simulink model "main_table_model"  (R2013a)
settings: Solver=ode3  StartTime=0.0  StopTime=Inf  FixedStep=1/30  RelTol=1e-3
undefined symbols (not defined in the file or in its folder): gray, none, serial, strel, videoinput
libraries: simulink x5, visiontextngfix x2, visionsinks x2, instrumentlib x2, visionstatistics x1, imaqlib x1, visionmorphops x1
settings Model: Creator=Michael  LastModifiedBy=nano

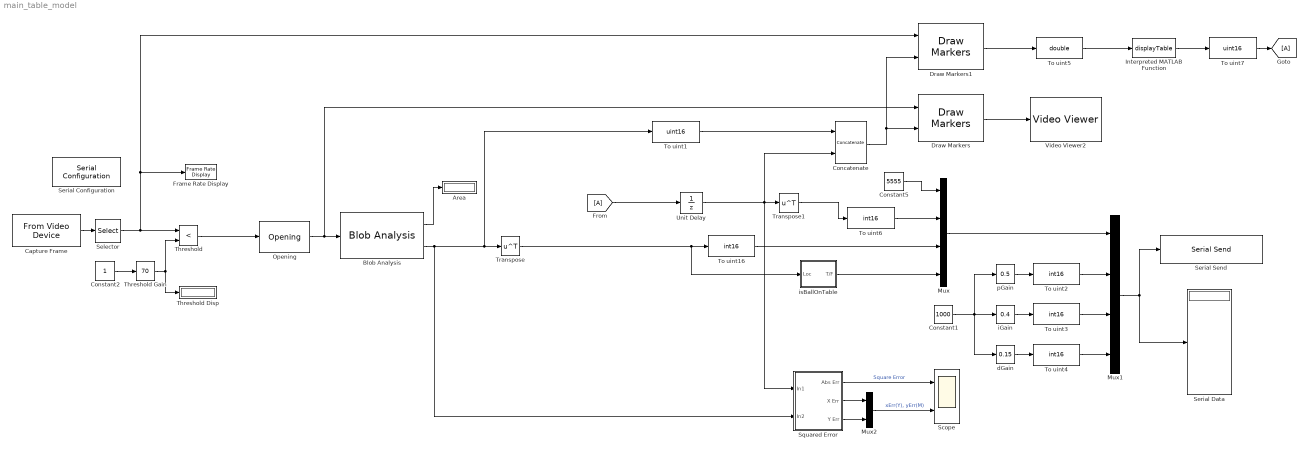
== system main_table_model ==
  Area : Display
  Blob Analysis : visionstatistics/Blob Analysis  Tag=vipblks_row_conv  area=on  centroid=on  bBox=off  majorAxis=off  minorAxis=off  angle=off  eccentricity=off  equivDiameterSq=off  extent=off  perimeter=off  maxBlobs=1  warnIfNumBlobsExceeded=off  isCount=off  useMinArea=on  minArea=50  useMaxArea=on  maxArea=1200  excludeBorderBlob=on  outDT=double  isOutVarDim=off  isFill=on  fillValues=-1  conn=8  isLabel=off  outputMode=Binary point scaling  outputWordLength=32  outputFracLength=16  firstCoeffMode=Binary point scaling  firstCoeffWordLength=16  firstCoeffFracLength=14  secondCoeffMode=Binary point scaling  secondCoeffWordLength=32  secondCoeffFracLength=16  accumMode=Binary point scaling  accumWordLength=32  accumFracLength=0  prodOutputMode=Binary point scaling  prodOutputWordLength=32  prodOutputFracLength=16  roundingMode=Floor  overflowMode=off
  Capture Frame : imaqlib/From Video Device  DeviceMenu=(none)  Device=winvideo 1 (HP Prem AF Webcam KQ245AA)  ObjConstructor=videoinput('winvideo', 1)  VideoFormatMenu=(none)  VideoFormat=MJPG_320x240  VideoSource=input1  ROIPosition=[0 0 240 320]  EnableHWTrigger=off  TriggerConfiguration=none/none  SampleTime=1/30  OutputPortsMode=One multidimensional signal  DataType=uint8  CanDoHWTrigger=no  ReturnedColorSpace=grayscale  BlockHandle=1913.0001  ROIWidth=320  ROIHeight=240  ROIColumn=0  ROIRow=0  EngXMLPath=C:\Program Files\MATLAB\R2013a\toolbox\imaq\imaq\private  DevXMLPath=C:\Program Files\MATLAB\R2013a\toolbox\imaq\imaqadaptors\win64  EngLibPath=C:\Program Files\MATLAB\R2013a\toolbox\imaq\imaqblks\imaqmex\win64  ColorSpace=grayscale  BayerSensorAlignment=grbg
  Concatenate : Concatenate  Mode=Multidimensional array
  Constant1 : Constant  Value=1000  OutDataTypeStr=double
  Constant2 : Constant  OutDataTypeStr=double
  Constant5 : Constant  Value=5555  OutDataTypeStr=int16
  Draw Markers : visiontextngfix/Draw Markers  shape=Plus  size=40  fill=off  fillClrSource=Specify via dialog  display=White  intensity=200  color=[150 0 0]  opacity=0.6  viewport=Entire image  antialiasing=off  inType=Obsolete  imagePorts=One multidimensional signal  prodOutputMode=Binary point scaling  prodOutputWordLength=32  prodOutputFracLength=14  memoryMode=Specify word length  memoryWordLength=16  memoryFracLength=15  roundingMode=Floor  overflowMode=off
  Draw Markers1 : visiontextngfix/Draw Markers  shape=Plus  size=40  fill=off  fillClrSource=Specify via dialog  display=White  intensity=200  color=[150 0 0]  opacity=0.6  viewport=Entire image  antialiasing=off  inType=Obsolete  imagePorts=One multidimensional signal  prodOutputMode=Binary point scaling  prodOutputWordLength=32  prodOutputFracLength=14  memoryMode=Specify word length  memoryWordLength=16  memoryFracLength=15  roundingMode=Floor  overflowMode=off
  Frame Rate Display : visionsinks/Frame Rate Display  UpdateRate=30
  Interpreted MATLAB Function : MATLABFcn  MATLABFcn=displayTable  Output1D=off
  Mux : Mux
  Mux1 : Mux
  Mux2 : Mux  Inputs=2
  Opening : visionmorphops/Opening  nhoodsrc=Specify via dialog  strel=strel('disk',7)
  Scope : Scope  NumInputPorts=2
      settings: TimeRange=20  YMin=0~-100  YMax=180~100  SaveName=PID_Error
  Selector : Selector  NumberOfDimensions=2  InputPortWidth=3  IndexOptions=Starting index (dialog),Starting index (dialog)  Indices=1,40  OutputSizes=240,240
  Serial Configuration : instrumentlib/Serial Configuration  Priority=-200000  ComPortMenu=COM7  ComPort=COM7  ObjConstructor=serial('COM7');  BaudRate=115200  DataBits=8  Parity=none  StopBits=1  FlowControl=none  Timeout=10  ByteOrder=LittleEndian
  Serial Data : Display
  Serial Send : instrumentlib/Serial Send  ComPortMenu=<Please select a port...>  ComPort=COM7  ObjConstructor=serial('COM7');  Terminator=<none>  EnableBlockingMode=on
  Squared Error : Subsystem
  Threshold : RelationalOperator  Operator=<  OutDataTypeStr=boolean  ZeroCross=off
  "Threshold Gain " : simulink/Math Operations/Slider Gain  low=0  gain=70  high=6070
  Threshold Disp : Display
  To uint1 : DataTypeConversion  OutDataTypeStr=uint16
  To uint{2..4,6,16} (5 alike) : DataTypeConversion  OutDataTypeStr=int16
  To uint5 : DataTypeConversion  OutDataTypeStr=double
  To uint7 : DataTypeConversion  OutDataTypeStr=uint16
  Transpose : Math  Operator=transpose  SaturateOnIntegerOverflow=on
  Transpose1 : Math  Operator=transpose  SaturateOnIntegerOverflow=on
  Unit Delay : UnitDelay  InitialCondition=[120, 120]  SampleTime=-1
  Video Viewer2 : visionsinks/Video Viewer  inputType=Obsolete7b  imagePorts=One multidimensional signal  useColorMap=off  colormapValue=gray(256)  specRange=off  minInputVal=0  maxInputVal=255  FigPos=[215 456 340 316]  AxisZoom=on  trueSizedOnce=off  OpenAtMdlStart=on  DefaultConfigurationName=vipscopes.VideoViewerScopeCfg
  dGain : simulink/Math Operations/Slider Gain  low=0  gain=0.15  high=1
  iGain : simulink/Math Operations/Slider Gain  low=0  gain=0.4  high=1
  isBallOnTable : Subsystem
  pGain : simulink/Math Operations/Slider Gain  low=0  gain=0.5  high=1
  wires:
  Opening/1 -> Blob Analysis/1, Draw Markers/1
  Transpose/1 -> isBallOnTable/1(Loc), To uint16/1
  Threshold/1 -> Opening/1
  To uint1/1 -> Concatenate/1
  Concatenate/1 -> Draw Markers1/2, Draw Markers/2
  Capture Frame/1 -> Selector/1
  isBallOnTable/1(T/F) -> Mux/4
  To uint16/1 -> Mux/3
  Transpose1/1 -> To uint6/1
  Constant5/1 -> Mux/1
  pGain/1 -> To uint2/1
  iGain/1 -> To uint3/1
  dGain/1 -> To uint4/1
  Constant1/1 -> dGain/1, iGain/1, pGain/1
  To uint2/1 -> Mux1/2
  To uint3/1 -> Mux1/3
  To uint4/1 -> Mux1/4
  Constant2/1 -> "Threshold Gain "/1
  "Threshold Gain "/1 -> Threshold/2, Threshold Disp/1
  [A] -> Unit Delay/1
  Selector/1 -> Frame Rate Display/1, Draw Markers1/1, Threshold/1
  Mux/1 -> Mux1/1
  Mux1/1 -> Serial Send/1, Serial Data/1
  Squared Error/1(Abs Err) -> Scope/1  "Square Error"
  To uint6/1 -> Mux/2
  Squared Error/2(X Err) -> Mux2/1
  Squared Error/3(Y Err) -> Mux2/2
  Mux2/1 -> Scope/2  "xErr(Y), yErr(M)"
  Blob Analysis/2 -> To uint1/1, Transpose/1, Squared Error/2(In2)
  Blob Analysis/1 -> Area/1
  Draw Markers1/1 -> To uint5/1
  Draw Markers/1 -> Video Viewer2/1
  To uint5/1 -> Interpreted MATLAB Function/1
  Interpreted MATLAB Function/1 -> To uint7/1
  To uint7/1 -> [A]
  Unit Delay/1 -> Concatenate/2, Squared Error/1(In1), Transpose1/1

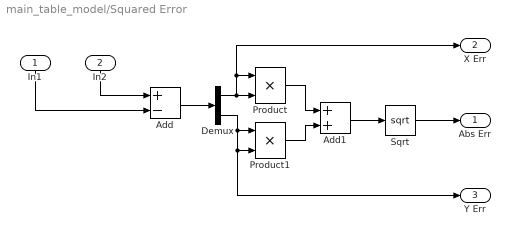
== system main_table_model/Squared Error ==
  In1 : Inport
  In2 : Inport  Port=2
  Add : Sum  Inputs=+-
  Add1 : Sum
  Demux : Demux  Outputs=2
  Product : Product
  Product1 : Product
  Sqrt : Sqrt  SaturateOnIntegerOverflow=on
  Abs Err : Outport
  X Err : Outport  Port=2
  Y Err : Outport  Port=3
  wires:
  Add1/1 -> Sqrt/1
  Demux/2 -> Y Err/1, Product1/2, Product1/1
  Product1/1 -> Add1/2
  Add/1 -> Demux/1
  Demux/1 -> X Err/1, Product/1, Product/2
  Product/1 -> Add1/1
  In1/1 -> Add/2
  In2/1 -> Add/1
  Sqrt/1 -> Abs Err/1

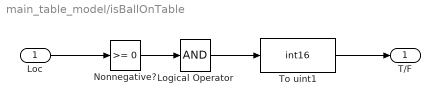
== system main_table_model/isBallOnTable ==
  Loc : Inport
  Logical Operator : Logic  Inputs=1  AllPortsSameDT=off  OutDataTypeStr=boolean
  Nonnegative? : simulink/Logic and Bit Operations/Compare To Zero  relop=>=  OutDataTypeStr=boolean  ZeroCross=off
  To uint1 : DataTypeConversion  OutDataTypeStr=int16
  T/F : Outport
  wires:
  Logical Operator/1 -> To uint1/1
  Nonnegative?/1 -> Logical Operator/1
  To uint1/1 -> T/F/1
  Loc/1 -> Nonnegative?/1
